simulink model "ProgettoTDL"  (R2021a)
settings: Solver=FixedStepAuto  StartTime=0.0  StopTime=100  FixedStep=0.001  RelTol=1e-3
model workspace (MAT data in the model file):
  A = Simulink.Parameter
  A.Value = [0  0  1  0; 0  0  0  1; 0  -60  0  -1.778; 4285.714  -4731.428  0  -13.206]
  A.DataType = 'auto'
  A.Dimensions = [4 4]
  B = Simulink.Parameter
  B.Value = [0; 0; 0.00222; 0.016508]
  B.DataType = 'auto'
  B.Dimensions = [4 1]
  C = Simulink.Parameter
  C.Value = [0 -60 0 -1.7778]
  C.DataType = 'auto'
  C.Dimensions = [1 4]
  D = Simulink.Parameter
  D.Value = 0.00222222222222
  D.DataType = 'auto'
  D.Dimensions = [1 1]
  E = Simulink.Parameter
  E.Value = [0; 0; 0; -4285.714]
  E.DataType = 'auto'
  E.Dimensions = [4 1]
  cmin = 800
  fmax = 3000
  k = 27000
  k0 = 38000
  kt = 300000
  ms = 450
  mu = 70
values from neighbouring files (symbols this model uses):
  A = [0 0 1 0; 0 0 0 1; 0 -60 0 -(16/9); (300000/70) -(33120/7) 0 -(832/63)]    [main_ScriptTDL.m]
  B = [0; 0; 0; -(300000/7)]    [main_ScriptTDL.m]
  C = [0 -60 0 -(16/9)]    [main_ScriptTDL.m]
  D = 0    [main_ScriptTDL.m]
  wr = 2*pi*data(2,i)/(3.6*200)    [main_ScriptTDL.m]    (also in parsenfile.m = 2*pi*data(2)/(3.6*200); parsenfilev2.m = 2*pi*data(2)/(3.6*200); parsenv3.m = 2*pi*data(2)/(3.6*200))
undefined symbols (not defined in the file or in its folder): ctr, Er, K, kr, u_mr
libraries: simulink x2, dspsrcs4 x1
settings Model: OrderedModelArguments=off  Creator=danis  LastModifiedBy=danis
settings SolverCC: AlgebraicLoopSolver=TrustRegion
settings DebuggingCC: SFMachineParentedDataDiag=warning

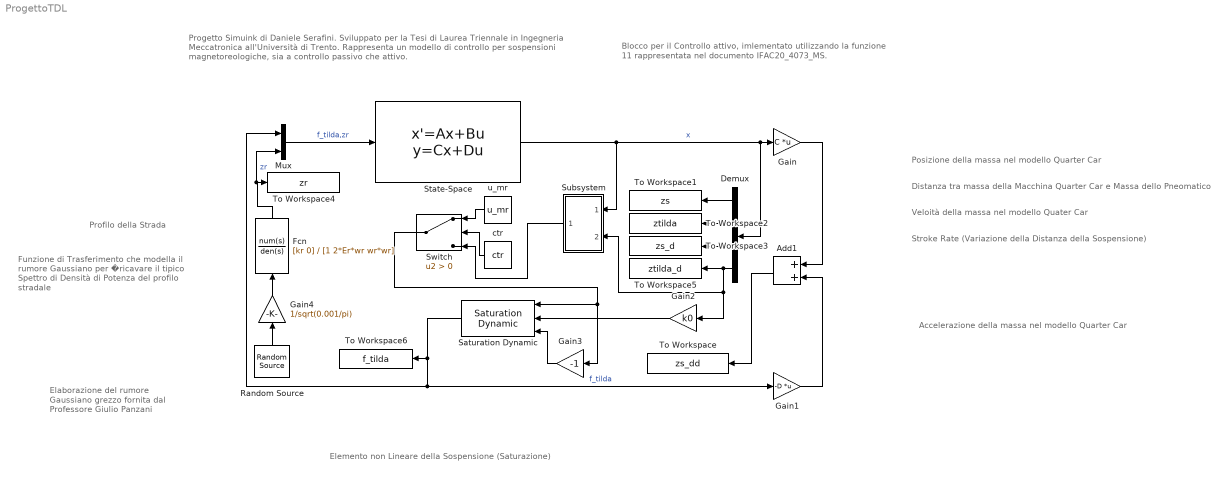
== system ProgettoTDL ==
  note: Elemento non Lineare della Sospensione (Saturazione)
  note: Stroke Rate (Variazione della Distanza della Sospensione)
  note: Distanza tra massa della Macchina Quarter Car e Massa dello Pneomatico
  note: Accelerazione della massa nel modello Quarter Car
  note: Veloità della massa nel modello Quater Car
  note: Posizione della massa nel modello Quarter Car
  note: Profilo della Strada
  note: Funzione di Trasferimento che modella il rumore Gaussiano per �ricavare il tipico Spettro di Densità di Potenza del profilo stradale
  note: Elaborazione del rumore Gaussiano grezzo fornita dal Professore Giulio Panzani
  note: Blocco per il Controllo attivo, imlementato utilizzando la funzione 11 rappresentata nel documento IFAC20_4073_MS.
  note: Progetto Simuink di Daniele Serafini. Sviluppato per la Tesi di Laurea Triennale in Ingegneria Meccatronica all'Università di Trento.
      | Rappresenta un modello di controllo per sospensioni magnetoreologiche, sia a controllo passivo che attivo.
  Add1 : Sum
  Demux : Demux
  Fcn : TransferFcn  Numerator=[kr 0]  Denominator=[1 2*Er*wr wr*wr]
  Gain : Gain  Gain=C  Multiplication=Matrix(K*u)
  Gain1 : Gain  Gain=-D  Multiplication=Matrix(K*u)
  Gain2 : Gain  Gain=k0
  Gain3 : Gain  Gain=-1
  Gain4 : Gain  Gain=1/sqrt(0.001/pi)
  Mux : Mux  Inputs=2
  Random Source : dspsrcs4/Random Source  SrcType=Gaussian  NormMethod=Ziggurat  CltLength=12  MinVal=0  MaxVal=1  MeanVal=0  VarVal=1  RepMode=Specify seed  rawSeed=1  IsInherit=off  SampMode=Discrete  SampTime=0.001  SampFrame=1  DataType=Double  OutComplex=Real  OutputFrames=off
  Saturation Dynamic : simulink/Discontinuities/Saturation Dynamic  OutMin=[]  OutMax=[]  OutDataTypeStr=Inherit: Same as second input  OutDataType=fixdt(1, 16)  OutScaling=2^-10  DoSatur=off
  State-Space : StateSpace  A=A  B=[-B E]  C=eye(4,4)  D=zeros(4,2)  InitialCondition=0
  Subsystem : Subsystem
  Switch : Switch  Criteria=u2 > Threshold
  To Workspace : ToWorkspace  VariableName=zs_dd  SampleTime=-1
      settings: Save2DSignal=2-D array (concatenate along first dimension)
  To Workspace1 : ToWorkspace  VariableName=zs  SampleTime=-1
      settings: Save2DSignal=2-D array (concatenate along first dimension)
  To Workspace2 : ToWorkspace  VariableName=ztilda  SampleTime=-1
      settings: Save2DSignal=2-D array (concatenate along first dimension)
  To Workspace3 : ToWorkspace  VariableName=zs_d  SampleTime=-1
      settings: Save2DSignal=2-D array (concatenate along first dimension)
  To Workspace4 : ToWorkspace  VariableName=zr  SampleTime=-1
      settings: Save2DSignal=2-D array (concatenate along first dimension)
  To Workspace5 : ToWorkspace  VariableName=ztilda_d  SampleTime=-1
      settings: Save2DSignal=2-D array (concatenate along first dimension)
  To Workspace6 : ToWorkspace  VariableName=f_tilda  SampleTime=-1
      settings: Save2DSignal=2-D array (concatenate along first dimension)
  ctr : Constant  Value=ctr
  u_mr : Constant  Value=u_mr
  wires:
  Mux/1 -> State-Space/1  "f_tilda,zr"
  State-Space/1 -> Subsystem/1(In1), Gain/1, Demux/1  "x"
  Saturation Dynamic/1 -> To Workspace6/1, Gain1/1, Mux/1  "f_tilda"
  Fcn/1 -> Mux/2, To Workspace4/1  "zr"
  Add1/1 -> To Workspace/1
  Demux/4 -> Subsystem/2(In2), Gain2/1, To Workspace5/1
  Gain2/1 -> Saturation Dynamic/2
  Demux/2 -> To Workspace2/1
  Demux/1 -> To Workspace1/1
  Gain/1 -> Add1/1
  Gain1/1 -> Add1/2
  Gain3/1 -> Saturation Dynamic/3
  Demux/3 -> To Workspace3/1
  Gain4/1 -> Fcn/1
  Random Source/1 -> Gain4/1
  Switch/1 -> Gain3/1, Saturation Dynamic/1
  u_mr/1 -> Switch/1
  Subsystem/1(Out1) -> Switch/3
  ctr/1 -> Switch/2

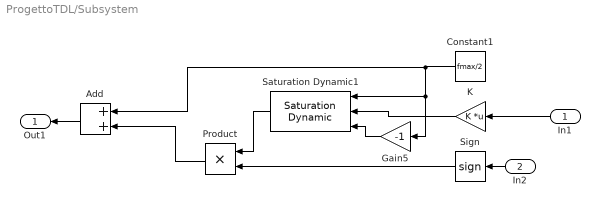
== system ProgettoTDL/Subsystem ==
  In1 : Inport
  In2 : Inport  Port=2
  Add : Sum
  Constant1 : Constant  Value=fmax/2
  Gain5 : Gain  Gain=-1
  K : Gain  Gain=K  Multiplication=Matrix(K*u)
  Product : Product
  Saturation Dynamic1 : simulink/Discontinuities/Saturation Dynamic  OutMin=[]  OutMax=[]  OutDataTypeStr=Inherit: Same as second input  OutDataType=fixdt(1, 16)  OutScaling=2^-10  DoSatur=off
  Sign : Signum
  Out1 : Outport
  wires:
  Add/1 -> Out1/1
  K/1 -> Saturation Dynamic1/2
  Gain5/1 -> Saturation Dynamic1/3
  Constant1/1 -> Gain5/1, Saturation Dynamic1/1, Add/1
  Sign/1 -> Product/2
  Saturation Dynamic1/1 -> Product/1
  Product/1 -> Add/2
  In2/1 -> Sign/1
  In1/1 -> K/1
